simulink model "betam"  (Simulink 7.2)
settings: Solver=ode45  StartTime=0.0  StopTime=10.0  RelTol=1e-3
settings Model: Creator=Dennis  LastModifiedBy=Dennis

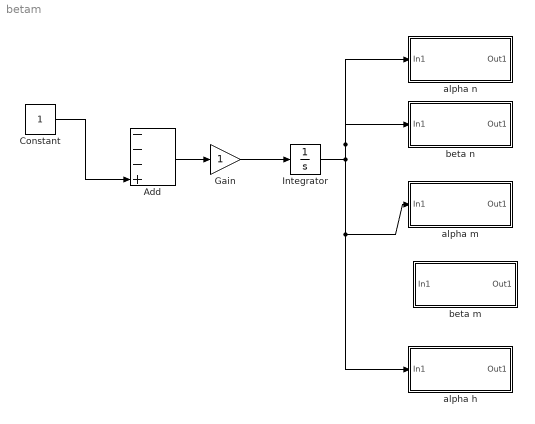
== system betam ==
  Add : Sum  Inputs=---+  OutDataType=sfix(16)  OutScaling=2^-10
  Constant : Constant  OutDataType=sfix(16)  OutScaling=2^0
  Gain : Gain  ParameterDataType=sfix(16)  ParameterScaling=2^0  OutDataType=sfix(16)  OutScaling=2^0
  Integrator : Integrator
  alpha h : Subsystem
  alpha m : Subsystem
  alpha n : Subsystem
  beta m : Subsystem
  beta n : Subsystem
  wires:
  Constant/1 -> Add/4
  Add/1 -> Gain/1
  Gain/1 -> Integrator/1
  Integrator/1 -> alpha m/1(In1), alpha h/1(In1), alpha n/1(In1), beta n/1(In1)

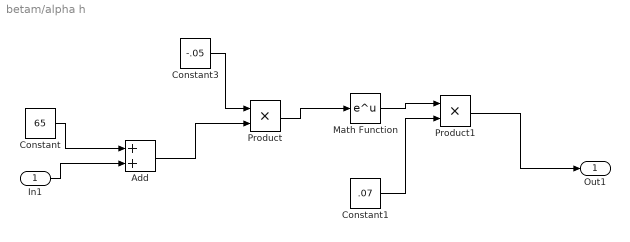
== system betam/alpha h ==
  In1 : Inport  OutDataType=sfix(16)  OutScaling=2^0
  Add : Sum  OutDataType=sfix(16)  OutScaling=2^-10
  Constant : Constant  Value=65  OutDataType=sfix(16)  OutScaling=2^0
  Constant1 : Constant  Value=.07  OutDataType=sfix(16)  OutScaling=2^0
  Constant3 : Constant  Value=-.05  OutDataType=sfix(16)  OutScaling=2^0
  Math Function : Math  OutDataType=sfix(16)  OutScaling=2^0  SaturateOnIntegerOverflow=on
  Product : Product  OutDataType=sfix(16)  OutScaling=2^0  RndMeth=Zero
  Product1 : Product  OutDataType=sfix(16)  OutScaling=2^0  RndMeth=Zero
  Out1 : Outport  OutDataType=sfix(16)  OutScaling=2^0
  wires:
  In1/1 -> Add/2
  Constant/1 -> Add/1
  Constant3/1 -> Product/1
  Add/1 -> Product/2
  Product/1 -> Math Function/1
  Math Function/1 -> Product1/1
  Constant1/1 -> Product1/2
  Product1/1 -> Out1/1

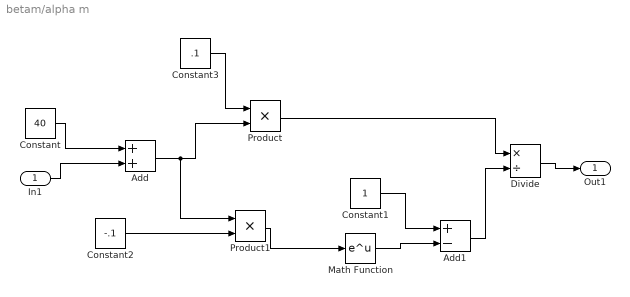
== system betam/alpha m ==
  In1 : Inport  OutDataType=sfix(16)  OutScaling=2^0
  Add : Sum  OutDataType=sfix(16)  OutScaling=2^-10
  Add1 : Sum  Inputs=+-  OutDataType=sfix(16)  OutScaling=2^-10
  Constant : Constant  Value=40  OutDataType=sfix(16)  OutScaling=2^0
  Constant1 : Constant  OutDataType=sfix(16)  OutScaling=2^0
  Constant2 : Constant  Value=-.1  OutDataType=sfix(16)  OutScaling=2^0
  Constant3 : Constant  Value=.1  OutDataType=sfix(16)  OutScaling=2^0
  Divide : Product  Inputs=*/  OutDataType=sfix(16)  OutScaling=2^-10
  Math Function : Math  OutDataType=sfix(16)  OutScaling=2^0  SaturateOnIntegerOverflow=on
  Product : Product  OutDataType=sfix(16)  OutScaling=2^0  RndMeth=Zero
  Product1 : Product  OutDataType=sfix(16)  OutScaling=2^0  RndMeth=Zero
  Out1 : Outport  OutDataType=sfix(16)  OutScaling=2^0
  wires:
  In1/1 -> Add/2
  Constant/1 -> Add/1
  Constant3/1 -> Product/1
  Add/1 -> Product/2, Product1/1
  Constant2/1 -> Product1/2
  Product1/1 -> Math Function/1
  Math Function/1 -> Add1/2
  Constant1/1 -> Add1/1
  Add1/1 -> Divide/2
  Product/1 -> Divide/1
  Divide/1 -> Out1/1

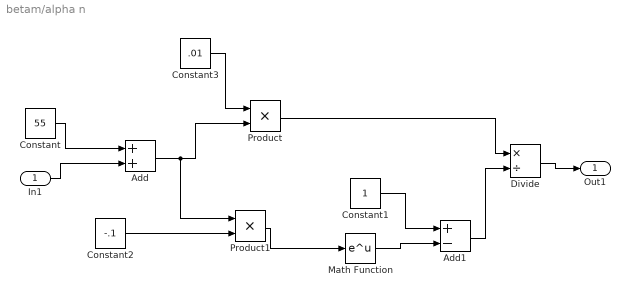
== system betam/alpha n ==
  In1 : Inport  OutDataType=sfix(16)  OutScaling=2^0
  Add : Sum  OutDataType=sfix(16)  OutScaling=2^-10
  Add1 : Sum  Inputs=+-  OutDataType=sfix(16)  OutScaling=2^-10
  Constant : Constant  Value=55  OutDataType=sfix(16)  OutScaling=2^0
  Constant1 : Constant  OutDataType=sfix(16)  OutScaling=2^0
  Constant2 : Constant  Value=-.1  OutDataType=sfix(16)  OutScaling=2^0
  Constant3 : Constant  Value=.01  OutDataType=sfix(16)  OutScaling=2^0
  Divide : Product  Inputs=*/  OutDataType=sfix(16)  OutScaling=2^-10
  Math Function : Math  OutDataType=sfix(16)  OutScaling=2^0  SaturateOnIntegerOverflow=on
  Product : Product  OutDataType=sfix(16)  OutScaling=2^0  RndMeth=Zero
  Product1 : Product  OutDataType=sfix(16)  OutScaling=2^0  RndMeth=Zero
  Out1 : Outport  OutDataType=sfix(16)  OutScaling=2^0
  wires:
  In1/1 -> Add/2
  Constant/1 -> Add/1
  Constant3/1 -> Product/1
  Add/1 -> Product/2, Product1/1
  Constant2/1 -> Product1/2
  Product1/1 -> Math Function/1
  Math Function/1 -> Add1/2
  Constant1/1 -> Add1/1
  Add1/1 -> Divide/2
  Product/1 -> Divide/1
  Divide/1 -> Out1/1

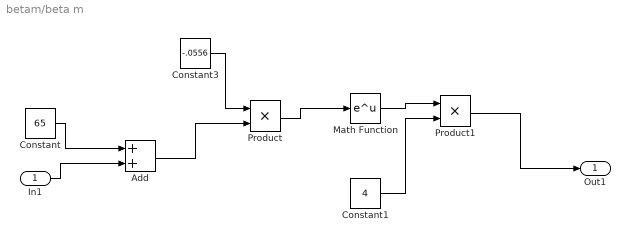
== system betam/beta m ==
  In1 : Inport  OutDataType=sfix(16)  OutScaling=2^0
  Add : Sum  OutDataType=sfix(16)  OutScaling=2^-10
  Constant : Constant  Value=65  OutDataType=sfix(16)  OutScaling=2^0
  Constant1 : Constant  Value=4  OutDataType=sfix(16)  OutScaling=2^0
  Constant3 : Constant  Value=-.0556  OutDataType=sfix(16)  OutScaling=2^0
  Math Function : Math  OutDataType=sfix(16)  OutScaling=2^0  SaturateOnIntegerOverflow=on
  Product : Product  OutDataType=sfix(16)  OutScaling=2^0  RndMeth=Zero
  Product1 : Product  OutDataType=sfix(16)  OutScaling=2^0  RndMeth=Zero
  Out1 : Outport  OutDataType=sfix(16)  OutScaling=2^0
  wires:
  In1/1 -> Add/2
  Constant/1 -> Add/1
  Constant3/1 -> Product/1
  Add/1 -> Product/2
  Product/1 -> Math Function/1
  Math Function/1 -> Product1/1
  Constant1/1 -> Product1/2
  Product1/1 -> Out1/1

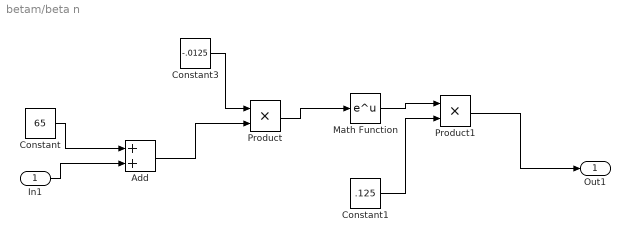
== system betam/beta n ==
  In1 : Inport  OutDataType=sfix(16)  OutScaling=2^0
  Add : Sum  OutDataType=sfix(16)  OutScaling=2^-10
  Constant : Constant  Value=65  OutDataType=sfix(16)  OutScaling=2^0
  Constant1 : Constant  Value=.125  OutDataType=sfix(16)  OutScaling=2^0
  Constant3 : Constant  Value=-.0125  OutDataType=sfix(16)  OutScaling=2^0
  Math Function : Math  OutDataType=sfix(16)  OutScaling=2^0  SaturateOnIntegerOverflow=on
  Product : Product  OutDataType=sfix(16)  OutScaling=2^0  RndMeth=Zero
  Product1 : Product  OutDataType=sfix(16)  OutScaling=2^0  RndMeth=Zero
  Out1 : Outport  OutDataType=sfix(16)  OutScaling=2^0
  wires:
  In1/1 -> Add/2
  Constant/1 -> Add/1
  Constant3/1 -> Product/1
  Add/1 -> Product/2
  Product/1 -> Math Function/1
  Math Function/1 -> Product1/1
  Constant1/1 -> Product1/2
  Product1/1 -> Out1/1
